simulink library "variableBuoyancy_ul"  (R2018b)
settings: Solver=VariableStepAuto  StartTime=0.0  StopTime=10.0  RelTol=1e-3
undefined symbols (not defined in the file): h, vol
libraries: dspstat3 x1
settings Model: Creator=Erin B  LastModifiedBy=mcobb

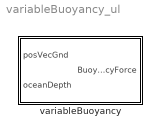
== system variableBuoyancy_ul ==
  variableBuoyancy : Subsystem  mask{vol=vol, h=h, rho=0, grav=0}
      mask prompts: vol "Volume"; h "Height of Object"; rho "Density"; grav "Gravity"

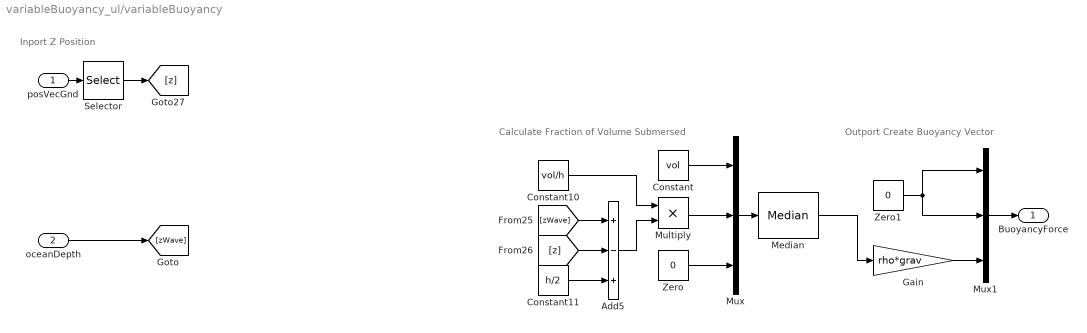
== system variableBuoyancy_ul/variableBuoyancy ==
  note: Inport Z Position
  note: Outport Create Buoyancy Vector
  note: Calculate Fraction of Volume Submersed
  posVecGnd : Inport
  oceanDepth : Inport  Port=2
  Add5 : Sum  Inputs=+-+
  Constant : Constant  Value=vol
  Constant10 : Constant  Value=vol/h
  Constant11 : Constant  Value=h/2
  Gain : Gain  Gain=rho*grav
  Median : dspstat3/Median  sortAlg=Quick sort  directionMode=Each column  dimension=1  roundingMode=Floor  overflowMode=off  accumDataTypeStr=Inherit: Same as product output  accumLastDataTypeStr=Inherit: Same as product output  outputDataTypeStr=Inherit: Same as accumulator  outputMin=[]  outputMax=[]  outputLastDataTypeStr=Inherit: Same as accumulator
      settings: SourceProductName=DSP System Toolbox  SourceProductBaseCode=DS  allowOverrides=off
  Multiply : Product
  Mux : Mux  Inputs=3
  Mux1 : Mux  Inputs=3
  Selector : Selector  InputPortWidth=3  IndexOptions=Index vector (dialog)  Indices=3  OutputSizes=1
  Zero : Constant  Value=0  OutDataTypeStr=Inherit: Inherit via back propagation
  Zero1 : Constant  Value=0  OutDataTypeStr=Inherit: Inherit via back propagation
  BuoyancyForce : Outport
  wires:
  Median/1 -> Gain/1
  Add5/1 -> Multiply/2
  [zWave] -> Add5/1
  Constant11/1 -> Add5/3
  [z] -> Add5/2
  Constant10/1 -> Multiply/1
  Mux/1 -> Median/1
  Constant/1 -> Mux/1
  Multiply/1 -> Mux/2
  Zero/1 -> Mux/3
  Gain/1 -> Mux1/3
  Mux1/1 -> BuoyancyForce/1
  Zero1/1 -> Mux1/1, Mux1/2
  posVecGnd/1 -> Selector/1
  Selector/1 -> [z]
  oceanDepth/1 -> [zWave]
